simulink model "sdrufreqcalib_rx"  (R2021a)
settings: Solver=FixedStepDiscrete  StartTime=0.0  StopTime=inf  RelTol=1e-3  EnableMultiTasking=on
PreLoadFcn:
  | platform = sdruExampleFindRadio;
  | prmFreqCalibRx = configureFreqCalibRx(platform, 900e6, 100);
  | clear platform
PostLoadFcn:
  | sdruExampleSetAvailableRadio;
InitFcn:
  | platform = get_param([gcs '/USRP Receiver'], 'Platform');
  | prmFreqCalibRx = configureFreqCalibRx(platform, 900e6, 100);
  | switch platform
  |   case 'X300'
  |     set_param([gcs,'/USRP Receiver'], 'masterClkRateX300','200e6');
  |   case 'X310'
  |     set_param([gcs,'/USRP Receiver'], 'masterClkRateX310','200e6');
  |   case 'N300'
  |     set_param([gcs,'/USRP Receiver'], 'masterClkRateN300','153.6e6');
  |   case 'N310'
  |     set_param([gcs,'/USRP Receiver'], 'masterClkRateN310','153.6e6');
  |   case 'N320/N321'
  |      set_param([gcs,'/USRP Receiver'], 'masterClkRateN320','200e6');
  | end
  | 
  | clear platform
libraries: sdrublksprivate x1, dspspect3 x1, commsdrhw_v2 x1
settings Model: SimulationMode=accelerator  Creator=The MathWorks, Inc.  LastModifiedBy=hymc
settings SolverCC: AlgebraicLoopSolver=TrustRegion
settings DataIOCC: LimitDataPoints=on  SaveFormat=Array  ReturnWorkspaceOutputs=off
settings OptimizationCC: ExpressionDepthLimit=2147483647  LifeSpan=inf
settings DebuggingCC: UnderspecifiedInitializationDetection=Classic  MergeDetectMultiDrivingBlocksExec=none  SolverPrmCheckMsg=warning  ParameterPrecisionLossMsg=none  FcnCallInpInsideContextMsg=warning  AllowSymbolicDim=off  StateNameClashWarn=warning  SFUnexpectedBacktrackingDiag=warning  SFNoUnconditionalDefaultTransitionDiag=warning  SFExecutionAtInitializationDiag=none  SFMachineParentedDataDiag=warning  ArithmeticOperatorsInVariantConditions=warning
settings HardwareCC: ProdBitPerPointer=32  ProdBitPerSizeT=32  ProdBitPerPtrDiffT=32  ProdLargestAtomicFloat=None  ProdIntDivRoundTo=Undefined  ProdEndianess=Unspecified  ProdWordSize=32  ProdHWDeviceType=32-bit Generic  TargetBitPerLong=64  TargetBitPerPointer=64  TargetBitPerSizeT=64  TargetBitPerPtrDiffT=64  TargetLongLongMode=on  TargetIntDivRoundTo=Zero  TargetEndianess=LittleEndian  TargetWordSize=64  TargetHWDeviceType=Generic->MATLAB Host Computer  ProdEqTarget=off
settings ModelReferenceCC: PropagateSignalLabelsOutOfModel=off
settings SFSimCC: SimUseLocalCustomCode=off  CustomCodeUndefinedFunction=UseInterfaceOnly
settings RTWCC: RTWUseLocalCustomCode=off
settings RTWCC: CustomSourceCode=|
  | #include<stdio.h>
  | #include<stdlib.h>
settings CodeAppCC: StateflowObjectComments=on
settings GRTTargetCC: TargetLangStandard=C89/C90 (ANSI)  CombineOutputUpdateFcns=off  GRTInterface=on
settings ConfigComp: CovMetricSettings=dw  CovSaveCumulativeToWorkspaceVar=on  CovSaveSingleToWorkspaceVar=on  CovExternalEMLEnable=off  CovSFcnEnable=off

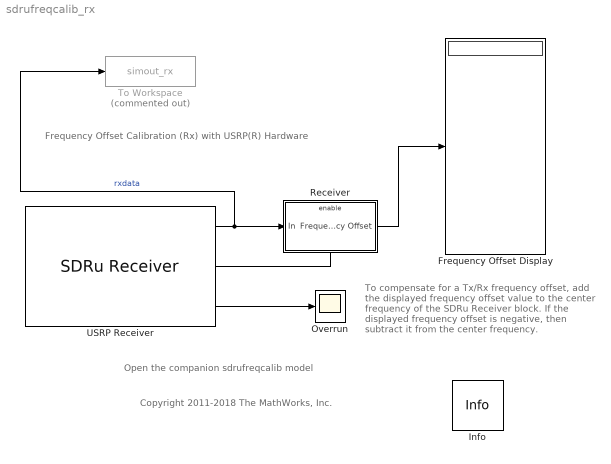
== system sdrufreqcalib_rx ==
  note: Frequency Offset Calibration (Rx)
      | with USRP(R) Hardware
  note: Open the companion sdrufreqcalib model
  note: Copyright 2011-2018 The MathWorks, Inc.
  note: To compensate for a Tx/Rx frequency offset,
      | add the displayed frequency offset value to the
      | center frequency of the SDRu Receiver block. If
      | the displayed frequency offset is negative, then
      | subtract it from the center frequency.
  Frequency Offset Display : Display
  Info : sdrublksprivate/Info  SystemSampleTime=-1  VariantActivationTime=update diagram  Latency=0  AutoFrameSizeCalculation=off
      settings: SourceProductBaseCode=USRP
  Overrun : Scope
  Receiver : Subsystem
      mask Display: disp('Receiver')
  To Workspace : ToWorkspace  Commented=on  VariableName=simout_rx  SaveFormat=Timeseries  SampleTime=-1
  USRP Receiver : commsdrhw_v2/SDRu Receiver  rxtx=rx  initializeIPAddress=0  devMap=10  USRP2_IP=192.168.10.2  USRP_IP_X300=192.168.1.22,192.168.1.23  USRP_IP_X310=192.168.1.25  USRP_IP_N300=192.168.10.2  USRP_IP_N310=192.168.10.2  USRP_IP_N320=192.168.10.2  USRP_serialNumB200=F4F58D  USRP_serialNumB210=3136D5F  platform=X300  prevPlatform=X300  lastIPAddressPopup=192.168.10.2  USRP_ID=192.168.1.22,192.168.1.23  LastIPAddress=192.168.10.2  IsTwinRXDaughterboard=off  EnableTwinRXPhaseSync=off  losrc=0  ChannelMapping=[1 2 3 4]  centerFrequencySrc=Dialog  centerFrequency=2.4e9  loOffsetSrc=Dialog  loOffset=0  gainSrc=Dialog  gain=23  PPSSource=External  EnableGPSLock=off  EnsureSyncGPSTime=off  clockSource=External  EnableRefLock=off  masterClkRateParam=200e6  masterClkRateB200=prmFreqCalibRx.MasterClockRate  masterClkRateB210=prmFreqCalibRx.MasterClockRate  masterClkRateX300=200e6  masterClkRateX310=200e6  masterClkRateN300=125e6  masterClkRateN310=125e6  masterClkRateN320=200e6  masterClkRate=100e6  masterClkRateTwinRX=200e6  decimInterpSrc=Dialog  decimInterpPort=512  lastDecimSource=Dialog  decimInterp=prmFreqCalibRx.DecimationFactor  USRP2_IP_NUM=[49 57 50 46 49 54 56 46 49 46 50 50 44 49 57 50 46 49 54 56 46 49 46 50 51]  sampleRate=200000  sampleTime=1000/200000000  TransportDataType=int16  overrunUnderrunPort=on  outputDatatype=double  frameLength=4096  HOST_DATA_PORT=0  HOST_CONTROL_PORT=0  USRP2_DATA_PORT=0  USRP2_CONTROL_PORT=0  bufferMode=Continuous streaming  EnableBurstMode=off  NumFramesInBurst=100
      settings: SourceProductBaseCode=USRP
  wires:
  USRP Receiver/1 -> To Workspace/1, Receiver/1(In)  "rxdata"
  USRP Receiver/2 -> Receiver/Enable
  USRP Receiver/3 -> Overrun/1
  Receiver/1(Frequency Offset) -> Frequency Offset Display/1

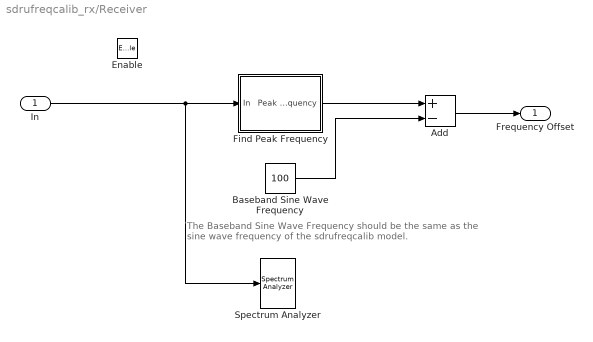
== system sdrufreqcalib_rx/Receiver ==
  note: The Baseband Sine Wave Frequency should be the same as
      | the sine wave frequency of the sdrufreqcalib model.
  In : Inport
  Enable : EnablePort
  Add : Sum  Inputs=+-
  Baseband Sine Wave Frequency : Constant  Value=100
  Find Peak Frequency : Subsystem
      mask Display: disp('Find Peak\nFrequency')
  Spectrum Analyzer : SpectrumAnalyzer
  Frequency Offset : Outport  VectorParamsAs1DForOutWhenUnconnected=off
  wires:
  In/1 -> Find Peak Frequency/1(In), Spectrum Analyzer/1
  Find Peak Frequency/1(Peak Frequency) -> Add/1
  Baseband Sine Wave Frequency/1 -> Add/2
  Add/1 -> Frequency Offset/1

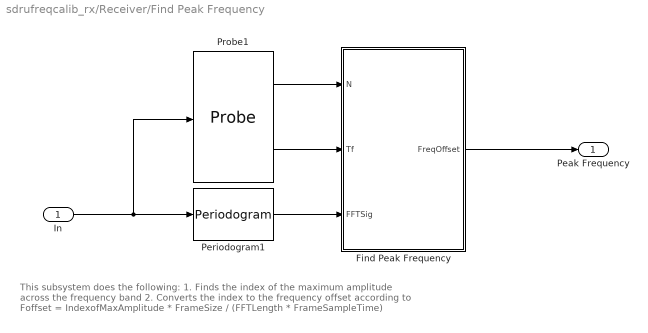
== system sdrufreqcalib_rx/Receiver/Find Peak Frequency ==
  note: This subsystem does the following:
      | 1.  Finds the index of the maximum amplitude across the frequency band
      | 2.  Converts the index to the frequency offset according to
      | Foffset = IndexofMaxAmplitude * FrameSize / (FFTLength * FrameSampleTime)
  In : Inport
  Find Peak Frequency : MATLAB Function  TreatAsAtomicUnit=on
  Periodogram1 : dspspect3/Periodogram  measurement=Power spectral density  wintype=Hamming  Rs=50  beta=5  winsamp=Symmetric  FFTImplementation=Auto  inheritFFT=off  fftsize=2048  navg=2  inheritTs=on  Ts=1
      settings: SourceProductBaseCode=DS
  Probe1 : Probe  ProbeComplexSignal=off
  Peak Frequency : Outport  VectorParamsAs1DForOutWhenUnconnected=off
  wires:
  Periodogram1/1 -> Find Peak Frequency/3(FFTSig)
  Probe1/1 -> Find Peak Frequency/1(N)
  Probe1/2 -> Find Peak Frequency/2(Tf)
  Find Peak Frequency/1(FreqOffset) -> Peak Frequency/1
  In/1 -> Periodogram1/1, Probe1/1

== matlab function sdrufreqcalib_rx/Receiver/Find Peak Frequency/Find Peak Frequency ==
  data: N input; FreqOffset output; Tf input; FFTSig input
function FreqOffset  = findpeakfreq(N, Tf, FFTSig)
% Find peak frequency
% N - frame size
% Tf - frame sample time
% FFTSig - result of FFT

%#codegen

FFTSize = length(FFTSig);
FFTSig = fftshift(FFTSig);
[~, maxIdx] = max(FFTSig); % Find index of max magnitude
OffsetIdx = maxIdx-1-FFTSize/2; % Convert to index symmetric with 0
Ts = Tf(1)/N; % Sample time
delta_f = 1/Ts/FFTSize; % Frequency resolution of FFT
FreqOffset = OffsetIdx*delta_f;% Map offset index back to frequency
